simulink model "vvvf"  (R2023a)
settings: Solver=ode23  StartTime=0.0  StopTime=9  MaxStep=5e-6  RelTol=1e-3
libraries: spsIGBTDiodeLib x6, simulink x2, spsAsynchronousMachineSIUnitsLib x1, spsTriangleGeneratorLib x1, slpidlib x1, spsDCVoltageSourceLib x1, spsVoltageMeasurementLib x1, spspowerguiLib x1
settings Model: SimulationMode=rapid-accelerator  Creator=搬砖工卢卡斯  LastModifiedBy=LabourerLucas
settings DebuggingCC: ParameterPrecisionLossMsg=none

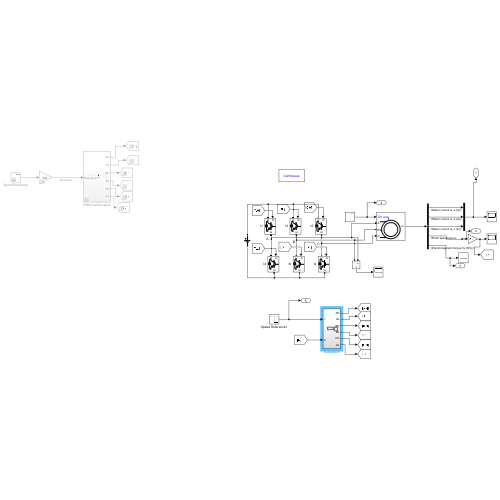
[thumbnail: Simulink's stored preview of the top-level diagram]
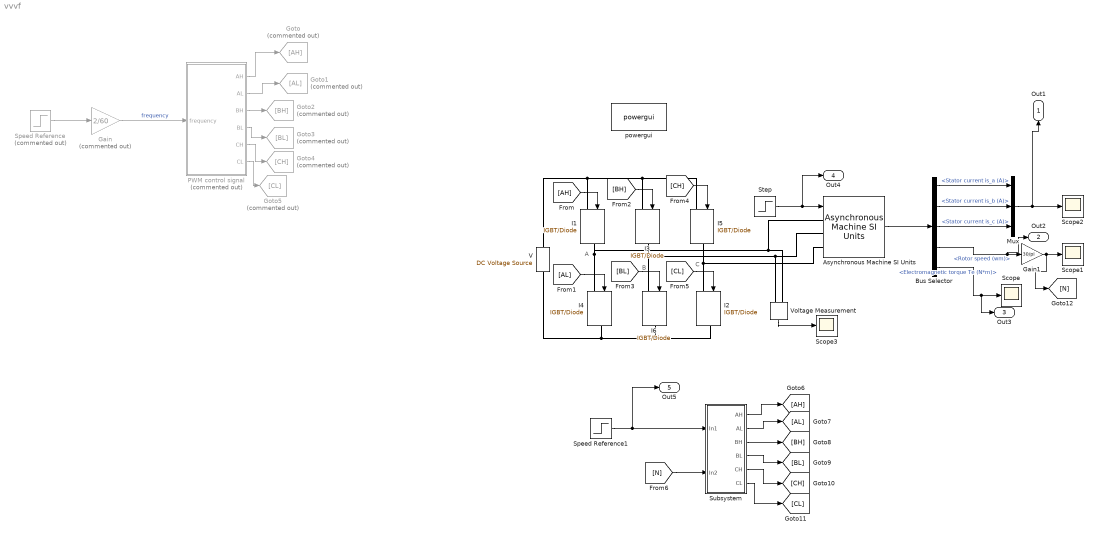
== system vvvf ==
  note: B
  note: C
  note: A
  Asynchronous Machine SI Units : spsAsynchronousMachineSIUnitsLib/Asynchronous Machine SI Units  RotorType=Squirrel-cage  PresetModel=No  MechanicalLoad=Torque Tm  ShowDetailedParameters=on  ReferenceFrame=Rotor  Units=SI  MeasurementBus=off  NominalParameters=[2200 200 50]  VoltageRatio=1  Stator=[0.877 0.0046]  Rotor=[1.47 0.0046]  Cage1=[0.4155 0.002066]  Cage2=[0.4168 0.0003495]  Lm=0.1608  Mechanical=[0.015 0 2]  PolePairs=2  InitialConditions=[1 0 0 0 0 0 0 0]  SimulateSaturation=off  Saturation=[14.03593122, 27.81365428, 53.79336849, 72.68890987, 97.98006896, 148.6815601, 215.7428561, 302.9841135, 428.7778367 ; 230, 322, 414, 460, 506, 552, 598, 644, 690]  LoadFlowParameters=1492000  TsPowergui=0  TsBlock=-1  IterativeModel=Trapezoidal non iterative  IterativeDiscreteModel=Trapezoidal non iterative  Pmec=1.492e+006
  Bus Selector : BusSelector  OutputSignals=Stator measurements.Stator current is_a (A),Stator measurements.Stator current is_b (A),Stator measurements.Stator current is_c (A),Mechanical.Rotor speed (wm),Mechanical.Electromagnetic torque Te (N*m)
  Gain : Gain  Commented=on  Gain=2/60
  Gain1 : Gain  Gain=30/pi
  Goto : Goto  Commented=on  GotoTag=AH
  Goto1 : Goto  Commented=on  GotoTag=AL
  Goto2 : Goto  Commented=on  GotoTag=BH
  Goto3 : Goto  Commented=on  GotoTag=BL
  Goto4 : Goto  Commented=on  GotoTag=CH
  Goto5 : Goto  Commented=on  GotoTag=CL
  I{1..6} (6 alike) : spsIGBTDiodeLib/IGBT//Diode  Ron=1e-3  Rs=1e5  Cs=inf  Measurements=off
  Mux : Mux  Inputs=3
  PWM control signal : Subsystem  Commented=on
  Scope{,1..3} (4 alike) : Scope
  Speed Reference : Step  Commented=on  Time=0  After=1500  SampleTime=0
  Speed Reference1 : Step  Time=3  Before=1430  After=1000  SampleTime=0
  Step : Step  Time=6  After=20  SampleTime=0
  Subsystem : Subsystem
  V : spsDCVoltageSourceLib/DC Voltage Source  Amplitude=500  Measurements=None
  Voltage Measurement : spsVoltageMeasurementLib/Voltage Measurement  PhasorSimulation=off  OutputType=Complex  PSBequivalent=0
  powergui : spspowerguiLib/powergui  Priority=1  SimulationMode=Continuous  SampleTime=1e-5  frequency=60  Iterations=50  frequencyindice=50  Pbase=100e6  ErrMax=1e-4  UnitsV=kV  UnitsW=MW  buscounter=0  FunctionMessages=off  echomessages=off  EnableUseOfTLC=off  CurrentSourceSwitches=off  DisableSnubberDevices=off  DisableRonSwitches=off  DisableVfSwitches=off  DisplayEquations=off  AutomaticDiscreteSolvers=off  SolverType=Tustin/Backward Euler (TBE)  Interpol=off  ExternalGateDelay=off  methode=off  Ts=100  x0status=blocks  SPID=on  SwTol=0  HookPort=off  NonlinearTolerance=1e-4  nMaxIteration=100  ContinueOnMaxIteration=off  RestoreLinks=warning  ResistiveCurrentMeasurement=off  Frange=[0:2:500]  Ylog=off  Xlog=on  ShowGrid=off  save=off  variable=ZData  structure=0  ZoomFFT=off  StartTime=0.0  cycles=1  DisplayStyle=1  fundamental=60  FreqAxis=off  MaxFrequency=1000  frequencyindicesteady=1  RmsSteady=1  display=off
  Out1 : Outport
  Out2 : Outport  Port=2
  Out3 : Outport  Port=3
  Out4 : Outport  Port=4
  Out5 : Outport  Port=5
  wires:
  Speed Reference/1 -> Gain/1
  Gain/1 -> PWM control signal/1(frequency)  "frequency"
  PWM control signal/1(AH) -> Goto/1
  PWM control signal/6(CL) -> Goto5/1
  PWM control signal/4(BL) -> Goto3/1
  PWM control signal/5(CH) -> Goto4/1
  PWM control signal/3(BH) -> Goto2/1
  PWM control signal/2(AL) -> Goto1/1
  [CH] -> I5/1
  [AH] -> I1/1
  [BH] -> I3/1
  [CL] -> I2/1
  [BL] -> I6/1
  [AL] -> I4/1
  Step/1 -> Out4/1, Asynchronous Machine SI Units/1
  Asynchronous Machine SI Units/1 -> Bus Selector/1
  Bus Selector/5 -> Out3/1, Scope/1  "<Electromagnetic torque Te (N*m)>"
  Bus Selector/4 -> Out2/1, Gain1/1  "<Rotor speed (wm)>"
  Gain1/1 -> Scope1/1, [N]
  Mux/1 -> Out1/1, Scope2/1
  Bus Selector/1 -> Mux/1  "<Stator current is_a (A)>"
  Bus Selector/2 -> Mux/2  "<Stator current is_b (A)>"
  Bus Selector/3 -> Mux/3  "<Stator current is_c (A)>"
  Voltage Measurement/1 -> Scope3/1
  Subsystem/1(AH) -> [AH]
  Subsystem/2(AL) -> [AL]
  Subsystem/3(BH) -> [BH]
  Subsystem/4(BL) -> [BL]
  Subsystem/5(CH) -> [CH]
  Subsystem/6(CL) -> [CL]
  Speed Reference1/1 -> Out5/1, Subsystem/1(In1)
  [N] -> Subsystem/2(In2)
  connections:
  I1/RConn1 -- Asynchronous Machine SI Units/LConn1 -- Voltage Measurement/LConn1 -- I4/LConn1
  I6/RConn1 -- V/LConn1 -- I4/RConn1 -- I2/RConn1
  I1/LConn1 -- V/RConn1 -- I5/LConn1 -- I3/LConn1
  I5/RConn1 -- Asynchronous Machine SI Units/LConn3 -- I2/LConn1
  I3/RConn1 -- Asynchronous Machine SI Units/LConn2 -- Voltage Measurement/LConn2 -- I6/LConn1

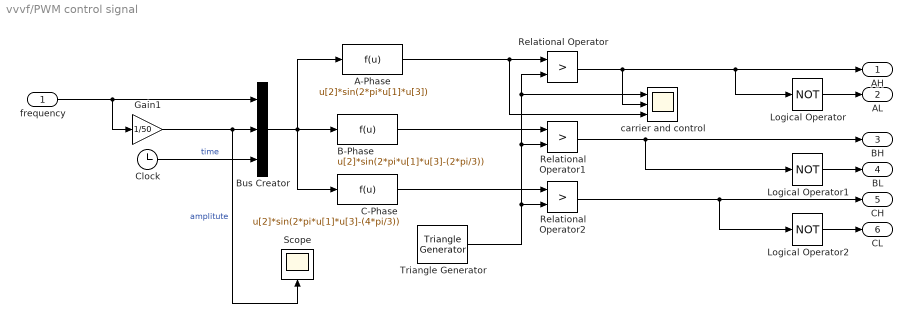
== system vvvf/PWM control signal ==
  frequency : Inport
  A-Phase : Fcn  Expr=u[2]*sin(2*pi*u[1]*u[3])
  B-Phase : Fcn  Expr=u[2]*sin(2*pi*u[1]*u[3]-(2*pi/3))
  Bus Creator : BusCreator  Inputs=3
  C-Phase : Fcn  Expr=u[2]*sin(2*pi*u[1]*u[3]-(4*pi/3))
  Clock : Clock
  Gain1 : Gain  Gain=1/50
  Logical Operator : Logic  Operator=NOT  IconShape=distinctive  AllPortsSameDT=off  OutDataTypeStr=boolean
  Logical Operator1 : Logic  Operator=NOT  IconShape=distinctive  AllPortsSameDT=off  OutDataTypeStr=boolean
  Logical Operator2 : Logic  Operator=NOT  IconShape=distinctive  AllPortsSameDT=off  OutDataTypeStr=boolean
  Relational Operator : RelationalOperator  Operator=>  OutDataTypeStr=boolean  InputSameDT=off
  Relational Operator1 : RelationalOperator  Operator=>  OutDataTypeStr=boolean  InputSameDT=off
  Relational Operator2 : RelationalOperator  Operator=>  OutDataTypeStr=boolean  InputSameDT=off
  Scope : Scope
  Triangle Generator : spsTriangleGeneratorLib/Triangle Generator  Freq=1000  Phase=90  Ts=0
  carrier and control : Scope  NumInputPorts=3
  AH : Outport
  AL : Outport  Port=2
  BH : Outport  Port=3
  BL : Outport  Port=4
  CH : Outport  Port=5
  CL : Outport  Port=6
  wires:
  frequency/1 -> Gain1/1, Bus Creator/1
  Relational Operator2/1 -> CH/1, Logical Operator2/1
  Bus Creator/1 -> C-Phase/1, B-Phase/1, A-Phase/1
  Relational Operator1/1 -> Logical Operator1/1, BH/1
  A-Phase/1 -> carrier and control/3, Relational Operator/1
  Relational Operator/1 -> carrier and control/2, AH/1, Logical Operator/1
  Triangle Generator/1 -> Relational Operator2/2, Relational Operator1/2, Relational Operator/2, carrier and control/1
  Clock/1 -> Bus Creator/3  "time"
  Gain1/1 -> Scope/1, Bus Creator/2  "amplitute"
  Logical Operator2/1 -> CL/1
  C-Phase/1 -> Relational Operator2/1
  Logical Operator/1 -> AL/1
  B-Phase/1 -> Relational Operator1/1
  Logical Operator1/1 -> BL/1

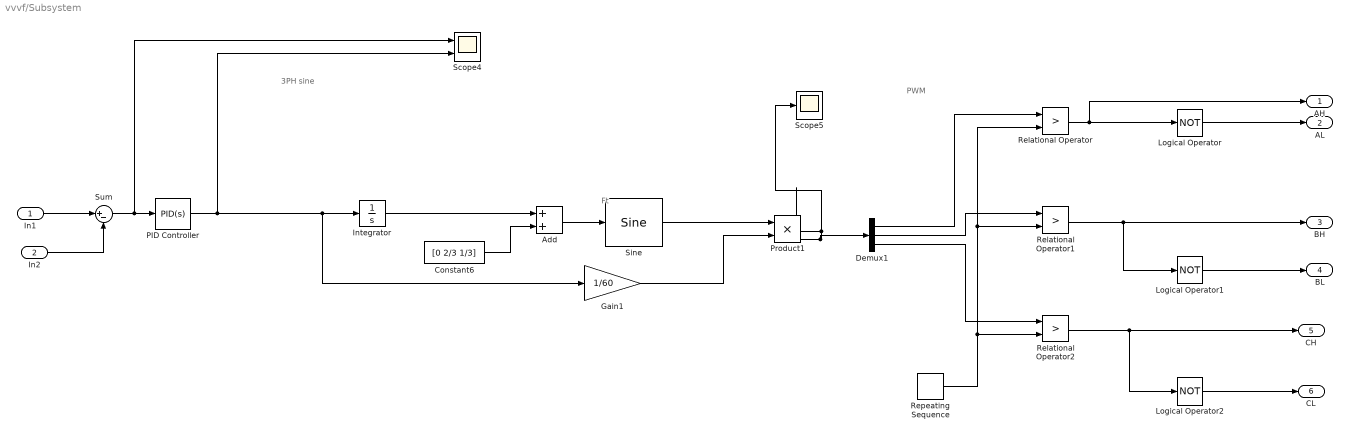
== system vvvf/Subsystem ==
  note: PWM
  note: 3PH sine
  note: Ft
  In1 : Inport
  In2 : Inport  Port=2
  Add : Sum
  Constant6 : Constant  Value=[0 2/3 1/3]
  Demux1 : Demux  Outputs=3
  Gain1 : Gain  Gain=1/60
  Integrator : Integrator
  Logical Operator : Logic  Operator=NOT  IconShape=distinctive  AllPortsSameDT=off  OutDataTypeStr=boolean
  Logical Operator1 : Logic  Operator=NOT  IconShape=distinctive  AllPortsSameDT=off  OutDataTypeStr=boolean
  Logical Operator2 : Logic  Operator=NOT  IconShape=distinctive  AllPortsSameDT=off  OutDataTypeStr=boolean
  PID Controller : slpidlib/PID Controller  Controller=PID  Form=Parallel  TimeDomain=Continuous-time  UseExternalTs=off  SampleTime=-1  IntegratorMethod=Forward Euler  FilterMethod=Forward Euler  ControllerParametersSource=internal  P=0.01  I=0.1  UseKiTs=off  D=0  N=100  UseFilter=on  TunerSelectOption=Transfer Function Based (PID Tuner App)  InitialConditionSource=internal  InitialConditionForIntegrator=0  InitialConditionForFilter=0  DifferentiatorICPrevScaledInput=0  ExternalReset=none  TrackingMode=off  Kt=1  LimitOutput=off  SatLimitsSource=internal  UpperSaturationLimit=inf  LowerSaturationLimit=-inf  LinearizeAsGain=on  AntiWindupMode=none  Kb=1  LimitIntegrator=off  UpperIntegratorSaturationLimit=inf  LowerIntegratorSaturationLimit=-inf  POutMin=[]  POutMax=[]  IOutMin=[]  IOutMax=[]  DOutMin=[]  DOutMax=[]  NOutMin=[]  NOutMax=[]  SumOutMin=[]  SumOutMax=[]  SaturationOutMin=[]  SaturationOutMax=[]  PParamMin=[]  PParamMax=[]  IParamMin=[]  IParamMax=[]  DParamMin=[]  DParamMax=[]  NParamMin=[]  NParamMax=[]  KbParamMin=[]  KbParamMax=[]  KtParamMin=[]  KtParamMax=[]  KbOutMin=[]  KbOutMax=[]  KtOutMin=[]  KtOutMax=[]  IntegratorOutMin=[]  IntegratorOutMax=[]  FilterOutMin=[]  FilterOutMax=[]  SumI1OutMin=[]  SumI1OutMax=[]  SumI2OutMin=[]  SumI2OutMax=[]  SumI3OutMin=[]  SumI3OutMax=[]  SumI4OutMin=[]  SumI4OutMax=[]  SumDOutMin=[]  SumDOutMax=[]  DifferentiatorOutMin=[]  DifferentiatorOutMax=[]  FilterDiffOutCoefMin=[]  FilterDiffOutCoefMax=[]  ReciprocalOutMin=[]  ReciprocalOutMax=[]  SumDenOutMin=[]  SumDenOutMax=[]  SumNumOutMin=[]  SumNumOutMax=[]  DivideOutMin=[]  DivideOutMax=[]  UdiffTsProdOutMin=[]  UdiffTsProdOutMax=[]  NTsProdOutMin=[]  NTsProdOutMax=[]  UintegralTsProdOutMin=[]  UintegralTsProdOutMax=[]  UngainTsProdOutMin=[]  UngainTsProdOutMax=[]  ClampingZeroOutDataTypeStr=Inherit: Inherit via back propagation  ClampingZeroOutMin=[]  ClampingZeroOutMax=[]  FilterDenConstantOutDataTypeStr=Inherit: Inherit via back propagation  FilterDenConstantOutMin=[]  FilterDenConstantOutMax=[]  PCopyOutDataTypeStr=Inherit: Inherit via back propagation  PCopyOutMin=[]  PCopyOutMax=[]  NCopyOutDataTypeStr=Inherit: Inherit via back propagation  NCopyOutMin=[]  NCopyOutMax=[]  IntegratorContinuousStateAttributes=''  IntegratorStateMustResolveToSignalObject=off  IntegratorRTWStateStorageClass=Auto  FilterContinuousStateAttributes=''  FilterStateMustResolveToSignalObject=off  FilterRTWStateStorageClass=Auto  ParallelPVariant=InternalParameters  IdealPVariant=Disabled  IVariant=InternalParameters  DVariant=InternalParameters  IntegratorVariant=Continuous  SatVariant=Disabled  AWVariant=Passthrough  PCopyVariant=Disabled  TRVariant=Disabled  FdbkBlocksVariant=Forward  IdealPFdbkVariant=Disabled  SatFdbkVariant=Disabled  DerivativeFilterVariant=ContFilter  NVariant=InternalParameters  NCopyVariant=Disabled  FilterICVariant=InternalICsFilter  IntegratorICVariant=InternalICs  ExternalResetVariant=Disabled  TRSumVariant=Passthrough  SumFdbkVariant=Disabled  SumVariant=Sum_PID  TsampFilterVariant=InternalTs  TsampNgainVariant=Passthrough  TsampIntegralVariant=Disabled_SignalSpec  ExternalSaturationOutDataTypeStr=Inherit: Same as second input
  Product1 : Product
  Relational Operator : RelationalOperator  Operator=>  OutDataTypeStr=boolean  InputSameDT=off
  Relational Operator1 : RelationalOperator  Operator=>  OutDataTypeStr=boolean  InputSameDT=off
  Relational Operator2 : RelationalOperator  Operator=>  OutDataTypeStr=boolean  InputSameDT=off
  Repeating Sequence : simulink/Sources/Repeating Sequence  rep_seq_t=[0 0.5/5000 1/5000]  rep_seq_y=[-1 1 -1]
  Scope4 : Scope  NumInputPorts=2
  Scope5 : Scope
  Sine : simulink/Lookup Tables/Sine  Formula=sin(2*pi*u)  NumDataPoints=(2^5)+1  OutputWordLength=16  InternalRulePriority=Speed
  Sum : Sum  Inputs=|+-
  AH : Outport
  AL : Outport  Port=2
  BH : Outport  Port=3
  BL : Outport  Port=4
  CH : Outport  Port=5
  CL : Outport  Port=6
  wires:
  Sum/1 -> Scope4/1, PID Controller/1
  Product1/1 -> Demux1/1, Scope5/1
  Relational Operator2/1 -> CH/1, Logical Operator2/1
  In2/1 -> Sum/2
  Logical Operator1/1 -> BL/1
  Relational Operator1/1 -> BH/1, Logical Operator1/1
  Logical Operator2/1 -> CL/1
  Logical Operator/1 -> AL/1
  In1/1 -> Sum/1
  Relational Operator/1 -> AH/1, Logical Operator/1
  Integrator/1 -> Add/1
  Add/1 -> Sine/1
  Constant6/1 -> Add/2
  Sine/1 -> Product1/1
  Gain1/1 -> Product1/2
  PID Controller/1 -> Gain1/1, Integrator/1, Scope4/2
  Demux1/2 -> Relational Operator1/1
  Repeating Sequence/1 -> Relational Operator1/2, Relational Operator/2, Relational Operator2/2
  Demux1/3 -> Relational Operator2/1
  Demux1/1 -> Relational Operator/1
